simulink model "A1_SIM3003"  (R2018b)
settings: Solver=VariableStepAuto  StartTime=0.0  StopTime=10.0  RelTol=1e-3
settings Model: Creator=student  LastModifiedBy=student

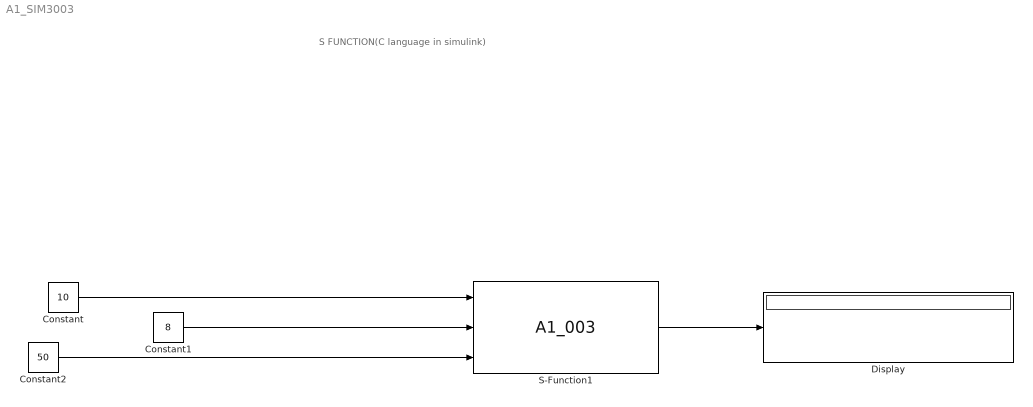
== system A1_SIM3003 ==
  note: S FUNCTION(C language in simulink)
  Constant : Constant  Value=10
  Constant1 : Constant  Value=8
  Constant2 : Constant  Value=50
  Display : Display
  S-Function1 : S-Function  FunctionName=A1_003  SFunctionDeploymentMode=off  EnableBusSupport=off
  wires:
  Constant/1 -> S-Function1/1
  Constant1/1 -> S-Function1/2
  S-Function1/1 -> Display/1
  Constant2/1 -> S-Function1/3
